simulink model "schema_di_controllo_nl_disturbi"  (R2023b)
settings: Solver=VariableStepAuto  StartTime=0.0  StopTime=1  RelTol=1e-3
undefined symbols (not defined in the file): C, k, u_e, WW, x_e
libraries: cstblocks x1
settings Model: Creator=guidocarnevale  LastModifiedBy=lverc

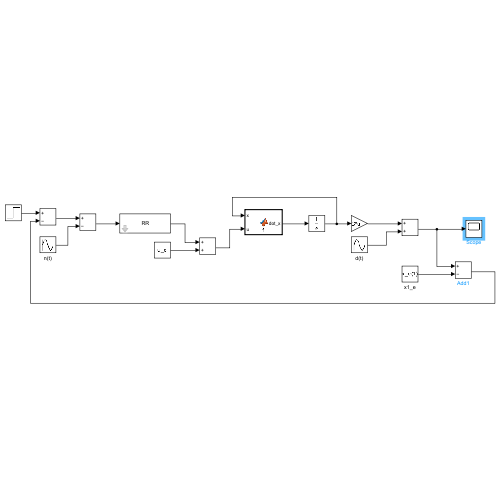
[thumbnail: Simulink's stored preview of the top-level diagram]
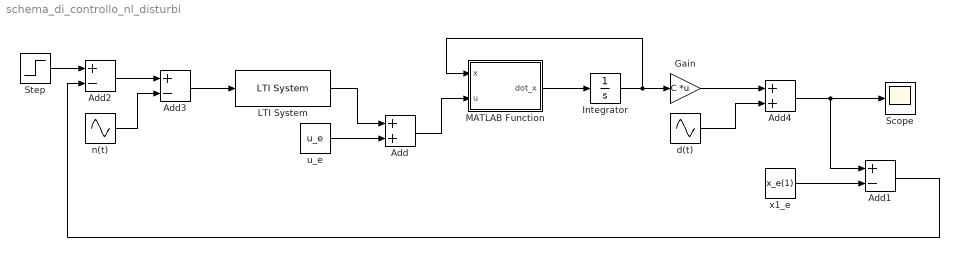
== system schema_di_controllo_nl_disturbi ==
  Add : Sum
  Add1 : Sum  Inputs=+-
  Add2 : Sum  Inputs=+-
  Add3 : Sum  Inputs=+-
  Add4 : Sum
  Gain : Gain  Gain=C  Multiplication=Matrix(K*u)
  Integrator : Integrator  InitialCondition=x_e
  LTI System : cstblocks/LTI System  sys=RR  IC=[]  PadeOrder=0
  MATLAB Function : MATLAB Function  TreatAsAtomicUnit=on
  Scope : Scope
  Step : Step  Time=0  After=WW  SampleTime=0
  d(t) : Sin  Amplitude=3  Frequency=0.01*k  SampleTime=0
  n(t) : Sin  Amplitude=3  Frequency=(10^5)*k  SampleTime=0
  u_e : Constant  Value=u_e
  x1_e : Constant  Value=x_e(1)
  wires:
  Add/1 -> MATLAB Function/2(u)
  u_e/1 -> Add/2
  MATLAB Function/1(dot_x) -> Integrator/1
  x1_e/1 -> Add1/2
  LTI System/1 -> Add/1
  Step/1 -> Add2/1
  Add1/1 -> Add2/2
  Add3/1 -> LTI System/1
  Add2/1 -> Add3/1
  n(t)/1 -> Add3/2
  Gain/1 -> Add4/1
  d(t)/1 -> Add4/2
  Add4/1 -> Scope/1, Add1/1
  Integrator/1 -> MATLAB Function/1(x), Gain/1

== matlab function schema_di_controllo_nl_disturbi/MATLAB Function ==
  data: x input; u input; dot_x output
function dot_x = f(x,u)

%Valori forniti da specifica
beta = 0.2;
k = 20;

J = @(theta) 2+0.5*cos(theta - 1) + 0.5*cos(2*theta +2) + 0.01*cos(3*theta + 1.5) + 0.01*cos(4*theta -2);

dot_x = zeros(2,1);

dot_x(1) = x(2);
dot_x(2) = -beta*x(2)/J(x(1)) + u/J(x(1)) - k*x(1)/J(x(1));
